simulink model "tut01"  (R2024a)
settings: Solver=VariableStepAuto  StartTime=0.0  StopTime=10.0  RelTol=1e-3
libraries: pil_lib x1
settings Model: Creator=User  LastModifiedBy=User
settings DataIOCC: LoadExternalInput=on  OutputSaveName=mdl_out  ReturnWorkspaceOutputsName=mdl_out  LoggingToFile=on  LoggingFileName=mdl_out.mat
settings OptimizationCC: DefaultParameterBehavior=Inlined  EnhancedBackFolding=on  PassReuseOutputArgsAs=Individual arguments  ZeroExternalMemoryAtStartup=off  ZeroInternalMemoryAtStartup=off  OptimizeBlockOrder=speed  DifferentSizesBufferReuse=on  OptimizationCustomize=off  EfficientTunableParamExpr=on
settings DebuggingCC: ParameterTunabilityLossMsg=error
settings SFSimCC: MATLABDynamicMemAlloc=off
settings RTWCC: Description=Embedded Coder  SystemTargetFile=ert.tlc  TemplateMakefile=ert_default_tmf  Toolchain=MinGW64 | gmake (64-bit Windows)
settings CodeAppCC: ForceParamTrailComments=on  IgnoreCustomStorageClasses=off  OperatorAnnotations=on  SimulinkDataObjDesc=on  SFDataObjDesc=on  InsertBlockDesc=on
settings ERTTargetCC: TargetLangStandard=C99 (ISO)  GenerateSampleERTMain=on  InlinedParameterPlacement=NonHierarchical  ERTCustomFileTemplate=example_file_process.tlc

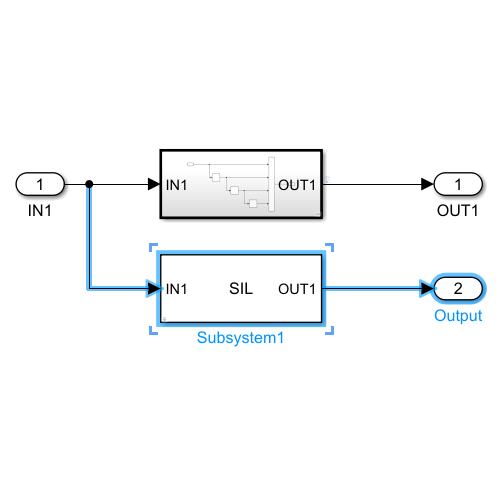
[thumbnail: Simulink's stored preview of the top-level diagram]
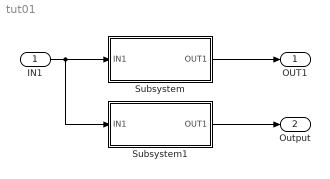
== system tut01 ==
  IN1 : Inport
  Subsystem : Subsystem  TreatAsAtomicUnit=on
  Subsystem1 : Subsystem  Tag=__SL_testing_harness_stub_  DialogController=pil_create_dialog  LoadFcn=|
      | try
      |    if ~strcmp(rtw.pil.getPILVersion, '24.1 (R2024a)_15')
      |       set_param(gcb, 'DialogController', '');
      |       set_param(gcb, 'DialogControllerArgs', '');
      |    end
      | catch e
      |       set_param(gcb, 'DialogController', '');
      |       set_param(gcb, 'DialogControllerArgs', '');
      | end
      mask help: PIL:pil:XILBlockMaskDesc
      mask Display: disp('SIL');
  OUT1 : Outport
  Output : Outport  Port=2
  wires:
  Subsystem/1(OUT1) -> OUT1/1
  IN1/1 -> Subsystem1/1(IN1), Subsystem/1(IN1)
  Subsystem1/1(OUT1) -> Output/1

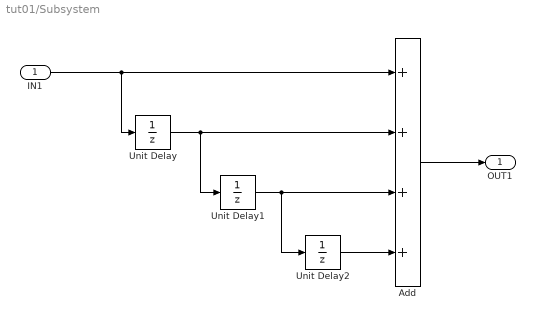
== system tut01/Subsystem ==
  IN1 : Inport
  Add : Sum  Inputs=++++
  Unit Delay : UnitDelay  SampleTime=-1  HasFrameUpgradeWarning=on
  Unit Delay1 : UnitDelay  SampleTime=-1  HasFrameUpgradeWarning=on
  Unit Delay2 : UnitDelay  SampleTime=-1  HasFrameUpgradeWarning=on
  OUT1 : Outport
  wires:
  IN1/1 -> Unit Delay/1, Add/1
  Unit Delay/1 -> Unit Delay1/1, Add/2
  Unit Delay1/1 -> Unit Delay2/1, Add/3
  Unit Delay2/1 -> Add/4
  Add/1 -> OUT1/1

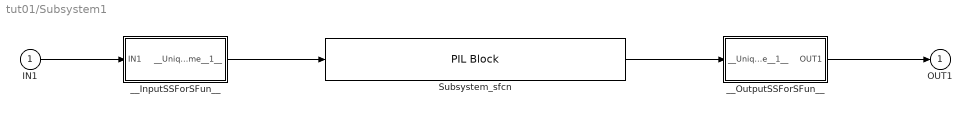
== system tut01/Subsystem1 ==
  IN1 : Inport
  Subsystem_sfcn : pil_lib/PIL Block  SimulationMode=SIL  IsTopModelPIL=off  CodeDir=Subsystem_ert_rtw  AnchorDir=D:\ME\Career\04.MBD\Tutorials\SIL_testing\tut01  ConfigName=Software-in-the-Loop (SIL)  XrelIsTopModelCode=on  XrelIsReusable=off  XrelDWorkNames={}  XrelDWorkTypes={}  XrelModelArgVals={}  XrelOrderedParamNames={}  XRelNonFiniteStyle=NONFINITE_UNUSED
  __InputSSForSFun__ : Subsystem
  __OutputSSForSFun__ : Subsystem
  OUT1 : Outport
  wires:
  __OutputSSForSFun__/1(OUT1) -> OUT1/1
  Subsystem_sfcn/1 -> __OutputSSForSFun__/1(__UniqueInportName__1__)
  __InputSSForSFun__/1(__UniqueOutportName__1__) -> Subsystem_sfcn/1
  IN1/1 -> __InputSSForSFun__/1(IN1)

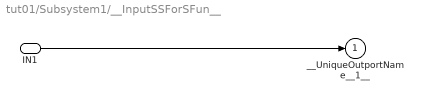
== system tut01/Subsystem1/__InputSSForSFun__ ==
  IN1 : Inport
  __UniqueOutportName__1__ : Outport
  wires:
  IN1/1 -> __UniqueOutportName__1__/1

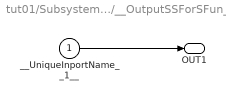
== system tut01/Subsystem1/__OutputSSForSFun__ ==
  __UniqueInportName__1__ : Inport
  OUT1 : Outport
  wires:
  __UniqueInportName__1__/1 -> OUT1/1
